simulink model "untitled"  (R2024a)
settings: Solver=VariableStepAuto  StartTime=0.0  StopTime=60  RelTol=1e-3
settings Model: Creator=Professional  LastModifiedBy=Professional

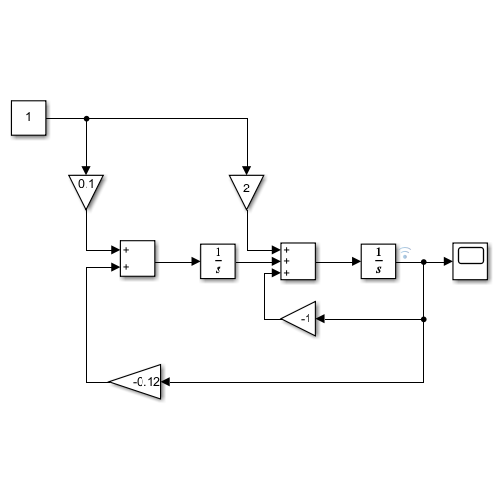
[thumbnail: Simulink's stored preview of the top-level diagram]
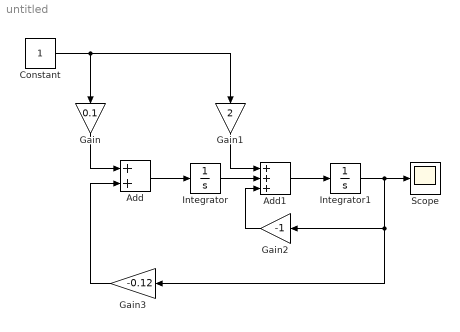
== system untitled ==
  Add : Sum
  Add1 : Sum  Inputs=+++
  Constant : Constant
  Gain : Gain  Gain=0.1
  Gain1 : Gain  Gain=2
  Gain2 : Gain  Gain=-1
  Gain3 : Gain  Gain=-0.12
  Integrator : Integrator
  Integrator1 : Integrator
  Scope : Scope
  wires:
  Constant/1 -> Gain1/1, Gain/1
  Gain/1 -> Add/1
  Add/1 -> Integrator/1
  Integrator/1 -> Add1/2
  Add1/1 -> Integrator1/1
  Integrator1/1 -> Scope/1, Gain3/1, Gain2/1
  Gain3/1 -> Add/2
  Gain2/1 -> Add1/3
  Gain1/1 -> Add1/1
